simulink model "OpenAUV_v1dist"  (R2025a)
settings: Solver=VariableStepAuto  StartTime=0.0  StopTime=80  RelTol=1e-3
InitFcn:
  | initialization
values from neighbouring files (symbols this model uses):
  cf_backward = 2.9e-5    (= 2.9e-05)    [initialization.m]
  cf_forward = 4.7e-5    (= 4.7e-05)    [initialization.m]
  D_L = diag([5.9341, 4.3172, 6.2491, 0.0199, 0.4611, 0.0698])    [initialization.m]
  D_Q = diag([19.374, 42.687, 51.0402, 0.0668, 1.9172, 1.1343])    [initialization.m]
  Delta = M / rho    (= 0.0185)    [initialization.m]
  g = 9.81    [initialization.m]
  Ib = diag([0.3432, 1.4483, 1.5047]) + Ib_added    [initialization.m]
  lin_vel_0 = [dot_x0 dot_y0 dot_z0]    [initialization.m]
  mass = M * eye(3) + M_a    [initialization.m]
  pos_0 = [x0 y0 z0]    [initialization.m]
  r_b_b = [-0.2; 0; 0.2]    [initialization.m]
  r_c_b = [0; 0; 0]    [initialization.m]
  rho = 1000    [initialization.m]
  Ts = 0.001    [initialization.m]
  w_bb_0 = [0 0 0]    [initialization.m]
undefined symbols (not defined in the file or in its folder): DiscIntNeverNeededParam
libraries: matrix_library x1
settings Model: Creator=fabioruggiero  LastModifiedBy=Acer
settings ModelReferenceCC: EnableRefExpFcnMdlSchedulingChecks=on
settings RTWCC: GPUComputeCapability=3.5

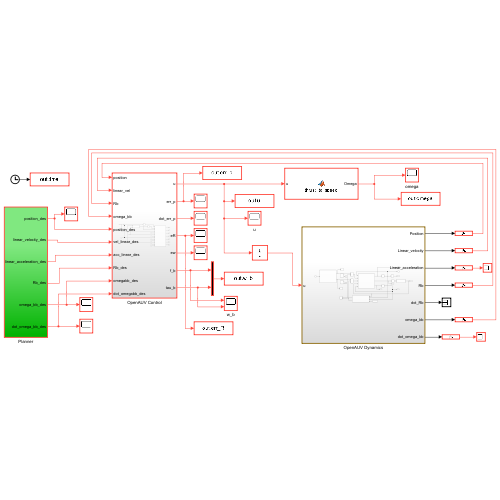
[thumbnail: Simulink's stored preview of the top-level diagram]
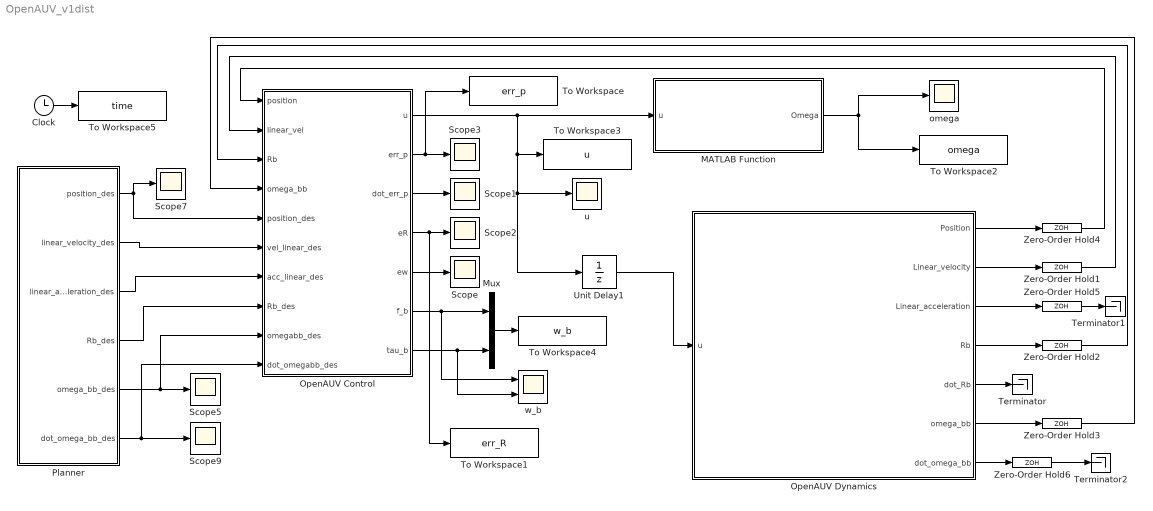
== system OpenAUV_v1dist ==
  Clock : Clock
  MATLAB Function : MATLAB Function  TreatAsAtomicUnit=on
  Mux : Mux  Inputs=2
  OpenAUV Control : Subsystem
  OpenAUV Dynamics : Subsystem
  Planner : Subsystem
  Scope{,1..3,5,7,9} (7 alike) : Scope
      Scope settings: Title=Angular Velocity errors  ActiveDisplayYMinimum=-1  ActiveDisplayYMaximum=1  YLabel=rad/s
      Scope1 settings: Title=Linear Velocity errors  ActiveDisplayYMinimum=-0.042668  ActiveDisplayYMaximum=0.038422  YLabel=m/s
      Scope2 settings: Title=Orientation error  ActiveDisplayYMinimum=-0.013334  ActiveDisplayYMaximum=0.012271
      Scope3 settings: Title=Position errors  ActiveDisplayYMinimum=-0.050218  ActiveDisplayYMaximum=0.073227  YLabel=m  DataLoggingVariableName=ScopeData2
      Scope5 settings: ActiveDisplayYMinimum=-0.15883  ActiveDisplayYMaximum=0.31625
      Scope7 settings: ActiveDisplayYMinimum=-4.625  ActiveDisplayYMaximum=1.625  DataLoggingVariableName=ScopeData2
      Scope9 settings: ActiveDisplayYMinimum=-0.05769  ActiveDisplayYMaximum=0.05769  DataLoggingVariableName=ScopeData2
  Terminator : Terminator
  Terminator1 : Terminator
  Terminator2 : Terminator
  To Workspace : ToWorkspace  VariableName=err_p  SaveFormat=Structure With Time  SampleTime=-1
  To Workspace1 : ToWorkspace  VariableName=err_R  SaveFormat=Structure With Time  SampleTime=-1
  To Workspace2 : ToWorkspace  VariableName=omega  SaveFormat=Structure With Time  SampleTime=-1
  To Workspace3 : ToWorkspace  VariableName=u  SaveFormat=Structure With Time  SampleTime=-1
  To Workspace4 : ToWorkspace  VariableName=w_b  SaveFormat=Structure With Time  SampleTime=-1
  To Workspace5 : ToWorkspace  VariableName=time  SaveFormat=Structure With Time  SampleTime=Ts
  Unit Delay1 : UnitDelay  InitialCondition=1.952815847891130e+05*ones(8,1)  SampleTime=-1
  Zero-Order Hold{1..6} (6 alike) : ZeroOrderHold  SampleTime=Ts
  omega : Scope
      settings: ActiveDisplayYMinimum=-1  ActiveDisplayYMaximum=1  DataLoggingVariableName=ScopeData3
  u : Scope
      settings: Title=u_w  ActiveDisplayYMinimum=-266.6856  ActiveDisplayYMaximum=244.3929  DataLoggingVariableName=ScopeData4
  w_b : Scope  NumInputPorts=2
      settings: Title=Control Forces  ActiveDisplayYMinimum=-17.0005  ActiveDisplayYMaximum=23.0413  YLabel=N
  wires:
  OpenAUV Dynamics/1(Position) -> Zero-Order Hold4/1
  OpenAUV Dynamics/2(Linear_velocity) -> Zero-Order Hold1/1
  OpenAUV Dynamics/4(Rb) -> Zero-Order Hold2/1
  OpenAUV Dynamics/6(omega_bb) -> Zero-Order Hold3/1
  Zero-Order Hold4/1 -> OpenAUV Control/1(position)
  OpenAUV Dynamics/5(dot_Rb) -> Terminator/1
  Planner/1(position_des) -> OpenAUV Control/5(position_des), Scope7/1
  OpenAUV Dynamics/3(Linear_acceleration) -> Zero-Order Hold5/1
  OpenAUV Dynamics/7(dot_omega_bb) -> Zero-Order Hold6/1
  Unit Delay1/1 -> OpenAUV Dynamics/1(u)
  Planner/4(Rb_des) -> OpenAUV Control/8(Rb_des)
  Planner/5(omega_bb_des) -> OpenAUV Control/9(omegabb_des), Scope5/1
  Planner/6(dot_omega_bb_des) -> OpenAUV Control/10(dot_omegabb_des), Scope9/1
  Zero-Order Hold5/1 -> Terminator1/1
  Zero-Order Hold6/1 -> Terminator2/1
  Mux/1 -> To Workspace4/1
  OpenAUV Control/7(tau_b) -> w_b/2, Mux/2
  OpenAUV Control/6(f_b) -> w_b/1, Mux/1
  OpenAUV Control/4(eR) -> To Workspace1/1, Scope2/1
  OpenAUV Control/2(err_p) -> Scope3/1, To Workspace/1
  Zero-Order Hold1/1 -> OpenAUV Control/2(linear_vel)
  Zero-Order Hold2/1 -> OpenAUV Control/3(Rb)
  Zero-Order Hold3/1 -> OpenAUV Control/4(omega_bb)
  Planner/2(linear_velocity_des) -> OpenAUV Control/6(vel_linear_des)
  Planner/3(linear_acceleration_des) -> OpenAUV Control/7(acc_linear_des)
  OpenAUV Control/3(dot_err_p) -> Scope1/1
  OpenAUV Control/5(ew) -> Scope/1
  Clock/1 -> To Workspace5/1
  MATLAB Function/1(Omega) -> To Workspace2/1, omega/1
  OpenAUV Control/1(u) -> MATLAB Function/1(u), Unit Delay1/1, u/1, To Workspace3/1

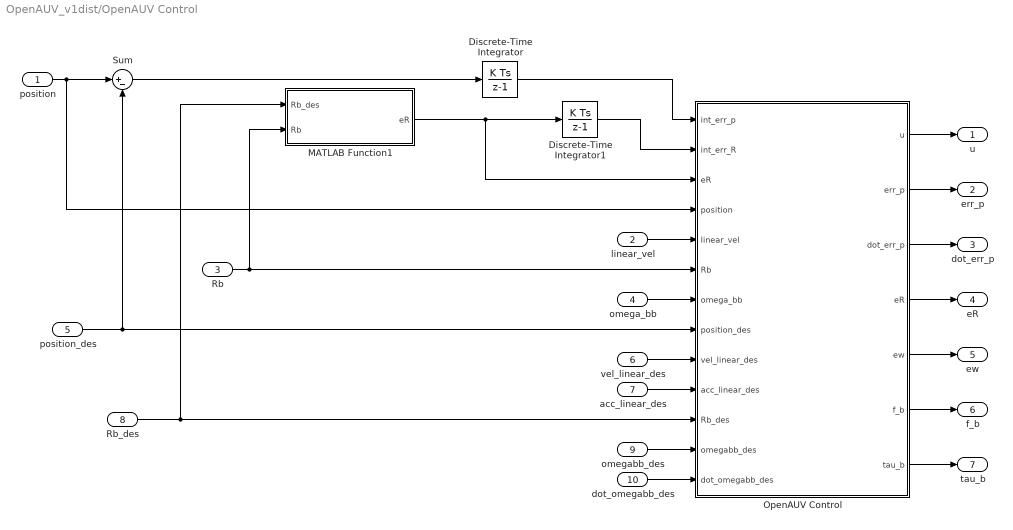
== system OpenAUV_v1dist/OpenAUV Control ==
  position : Inport
  linear_vel : Inport  Port=2
  Rb : Inport  Port=3
  omega_bb : Inport  Port=4
  position_des : Inport  Port=5
  vel_linear_des : Inport  Port=6
  acc_linear_des : Inport  Port=7
  Rb_des : Inport  Port=8
  omegabb_des : Inport  Port=9
  dot_omegabb_des : Inport  Port=10
  Discrete-Time Integrator : DiscreteIntegrator  SampleTime=Ts  UpperSaturationLimit=1.44  LowerSaturationLimit=-1.44  ICPrevOutput=DiscIntNeverNeededParam  ICPrevScaledInput=DiscIntNeverNeededParam
  Discrete-Time Integrator1 : DiscreteIntegrator  SampleTime=Ts  UpperSaturationLimit=1.44  LowerSaturationLimit=-1.44  ICPrevOutput=DiscIntNeverNeededParam  ICPrevScaledInput=DiscIntNeverNeededParam
  MATLAB Function1 : MATLAB Function  TreatAsAtomicUnit=on
  OpenAUV Control : MATLAB Function  TreatAsAtomicUnit=on
  Sum : Sum  Inputs=|+-
  u : Outport
  err_p : Outport  Port=2
  dot_err_p : Outport  Port=3
  eR : Outport  Port=4
  ew : Outport  Port=5
  f_b : Outport  Port=6
  tau_b : Outport  Port=7
  wires:
  OpenAUV Control/2(err_p) -> err_p/1
  vel_linear_des/1 -> OpenAUV Control/9(vel_linear_des)
  OpenAUV Control/3(dot_err_p) -> dot_err_p/1
  acc_linear_des/1 -> OpenAUV Control/10(acc_linear_des)
  OpenAUV Control/5(ew) -> ew/1
  dot_omegabb_des/1 -> OpenAUV Control/13(dot_omegabb_des)
  OpenAUV Control/4(eR) -> eR/1
  omegabb_des/1 -> OpenAUV Control/12(omegabb_des)
  OpenAUV Control/1(u) -> u/1
  Rb_des/1 -> MATLAB Function1/1(Rb_des), OpenAUV Control/11(Rb_des)
  position_des/1 -> Sum/2, OpenAUV Control/8(position_des)
  Sum/1 -> Discrete-Time Integrator/1
  MATLAB Function1/1(eR) -> OpenAUV Control/3("eR "), Discrete-Time Integrator1/1
  Discrete-Time Integrator/1 -> OpenAUV Control/1(int_err_p)
  Discrete-Time Integrator1/1 -> OpenAUV Control/2(int_err_R)
  position/1 -> OpenAUV Control/4(position), Sum/1
  linear_vel/1 -> OpenAUV Control/5(linear_vel)
  Rb/1 -> MATLAB Function1/2(Rb), OpenAUV Control/6(Rb)
  omega_bb/1 -> OpenAUV Control/7(omega_bb)
  OpenAUV Control/6(f_b) -> f_b/1
  OpenAUV Control/7(tau_b) -> tau_b/1

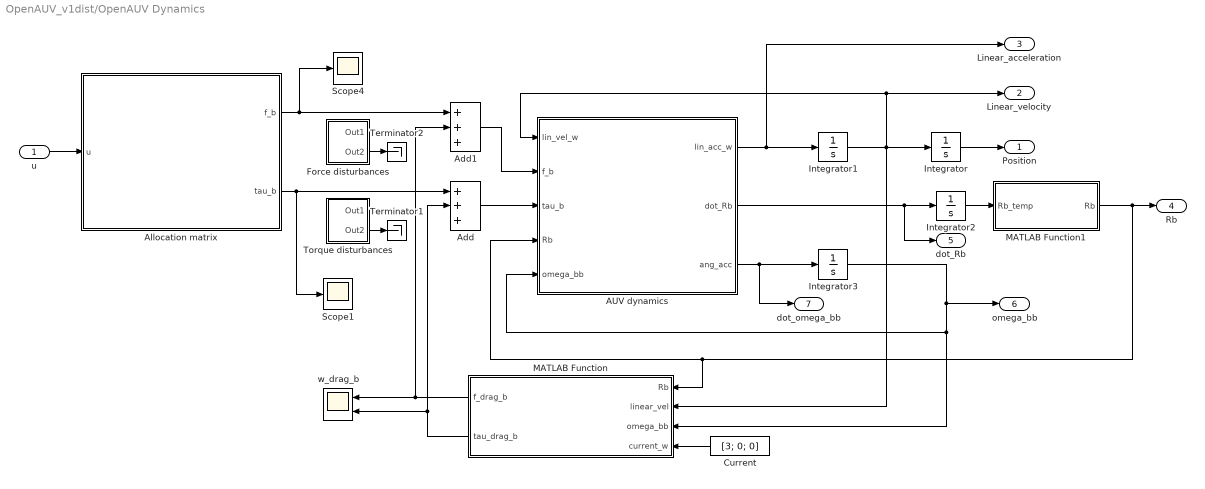
== system OpenAUV_v1dist/OpenAUV Dynamics ==
  u : Inport
  AUV dynamics : MATLAB Function  TreatAsAtomicUnit=on
  Add : Sum  Inputs=+++
  Add1 : Sum  Inputs=+++
  Allocation matrix : MATLAB Function  TreatAsAtomicUnit=on
  Current : Constant  Value=[3; 0; 0]
  Force disturbances : Subsystem
  Integrator : Integrator  InitialCondition=pos_0
  Integrator1 : Integrator  InitialCondition=lin_vel_0
  Integrator2 : Integrator  InitialCondition=[1 0 0; 0 1 0;0 0 1]
  Integrator3 : Integrator  InitialCondition=w_bb_0
  MATLAB Function : MATLAB Function  TreatAsAtomicUnit=on
  MATLAB Function1 : MATLAB Function  TreatAsAtomicUnit=on
  Scope1 : Scope
      settings: ActiveDisplayYMinimum=59.5491  ActiveDisplayYMaximum=72.8634  DataLoggingVariableName=ScopeData5
  Scope4 : Scope
      settings: ActiveDisplayYMinimum=-313.8933  ActiveDisplayYMaximum=214.6097  DataLoggingVariableName=ScopeData4
  Terminator1 : Terminator
  Terminator2 : Terminator
  Torque disturbances : Subsystem
  w_drag_b : Scope  NumInputPorts=2
      settings: Title=f_drag_b  ActiveDisplayYMinimum=-0.27226  ActiveDisplayYMaximum=1.5303  YLabel=N
  Position : Outport
  Linear_velocity : Outport  Port=2
  Linear_acceleration : Outport  Port=3
  Rb : Outport  Port=4
  dot_Rb : Outport  Port=5
  omega_bb : Outport  Port=6
  dot_omega_bb : Outport  Port=7
  wires:
  Integrator/1 -> Position/1
  AUV dynamics/3(ang_acc) -> dot_omega_bb/1, Integrator3/1
  Integrator3/1 -> MATLAB Function/3(omega_bb), AUV dynamics/5(omega_bb), omega_bb/1
  AUV dynamics/2(dot_Rb) -> dot_Rb/1, Integrator2/1
  MATLAB Function1/1(Rb) -> Rb/1, MATLAB Function/1(Rb), AUV dynamics/4(Rb)
  Integrator2/1 -> MATLAB Function1/1(Rb_temp)
  u/1 -> Allocation matrix/1(u)
  AUV dynamics/1(lin_acc_w) -> Linear_acceleration/1, Integrator1/1
  Add/1 -> AUV dynamics/3(tau_b)
  Add1/1 -> AUV dynamics/2(f_b)
  MATLAB Function/1(f_drag_b) -> w_drag_b/1, Add1/2
  MATLAB Function/2(tau_drag_b) -> w_drag_b/2, Add/2
  Current/1 -> MATLAB Function/4(current_w)
  Integrator1/1 -> Integrator/1, MATLAB Function/2(linear_vel), Linear_velocity/1, AUV dynamics/1(lin_vel_w)
  Allocation matrix/2(tau_b) -> Add/1, Scope1/1
  Allocation matrix/1(f_b) -> Scope4/1, Add1/1
  Force disturbances/2(Out2) -> Terminator2/1
  Torque disturbances/2(Out2) -> Terminator1/1

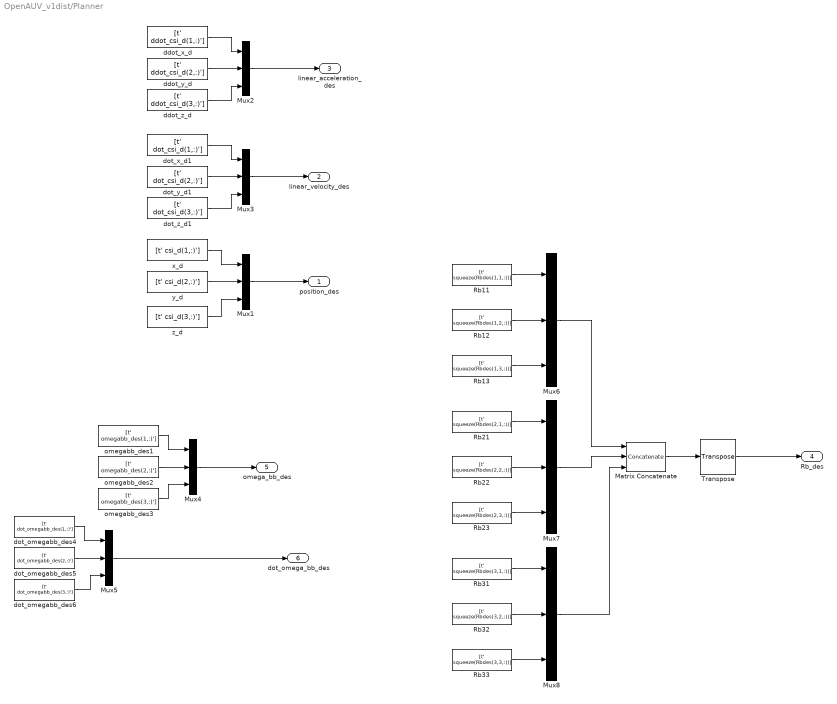
== system OpenAUV_v1dist/Planner ==
  Matrix Concatenate : Concatenate  NumInputs=3  Mode=Multidimensional array  ConcatenateDimension=2
  Mux{1..8} (8 alike) : Mux  Inputs=3
  Rb11 : FromWorkspace  VariableName=[t' squeeze(Rbdes(1,1,:))]  SampleTime=Ts
  Rb12 : FromWorkspace  VariableName=[t' squeeze(Rbdes(1,2,:))]  SampleTime=Ts
  Rb13 : FromWorkspace  VariableName=[t' squeeze(Rbdes(1,3,:))]  SampleTime=Ts
  Rb21 : FromWorkspace  VariableName=[t' squeeze(Rbdes(2,1,:))]  SampleTime=Ts
  Rb22 : FromWorkspace  VariableName=[t' squeeze(Rbdes(2,2,:))]  SampleTime=Ts
  Rb23 : FromWorkspace  VariableName=[t' squeeze(Rbdes(2,3,:))]  SampleTime=Ts
  Rb31 : FromWorkspace  VariableName=[t' squeeze(Rbdes(3,1,:))]  SampleTime=Ts
  Rb32 : FromWorkspace  VariableName=[t' squeeze(Rbdes(3,2,:))]  SampleTime=Ts
  Rb33 : FromWorkspace  VariableName=[t' squeeze(Rbdes(3,3,:))]  SampleTime=Ts
  Transpose : matrix_library/Transpose
  ddot_x_d : FromWorkspace  VariableName=[t' ddot_csi_d(1,:)']  SampleTime=Ts
  ddot_y_d : FromWorkspace  VariableName=[t' ddot_csi_d(2,:)']  SampleTime=Ts
  ddot_z_d : FromWorkspace  VariableName=[t' ddot_csi_d(3,:)']  SampleTime=Ts
  dot_omegabb_des4 : FromWorkspace  VariableName=[t' dot_omegabb_des(1,:)']  SampleTime=Ts
  dot_omegabb_des5 : FromWorkspace  VariableName=[t' dot_omegabb_des(2,:)']  SampleTime=Ts
  dot_omegabb_des6 : FromWorkspace  VariableName=[t' dot_omegabb_des(3,:)']  SampleTime=Ts
  dot_x_d1 : FromWorkspace  VariableName=[t' dot_csi_d(1,:)']  SampleTime=Ts
  dot_y_d1 : FromWorkspace  VariableName=[t' dot_csi_d(2,:)']  SampleTime=Ts
  dot_z_d1 : FromWorkspace  VariableName=[t' dot_csi_d(3,:)']  SampleTime=Ts
  omegabb_des1 : FromWorkspace  VariableName=[t' omegabb_des(1,:)']  SampleTime=Ts
  omegabb_des2 : FromWorkspace  VariableName=[t' omegabb_des(2,:)']  SampleTime=Ts
  omegabb_des3 : FromWorkspace  VariableName=[t' omegabb_des(3,:)']  SampleTime=Ts
  x_d : FromWorkspace  VariableName=[t' csi_d(1,:)']  SampleTime=Ts
  y_d : FromWorkspace  VariableName=[t' csi_d(2,:)']  SampleTime=Ts
  z_d : FromWorkspace  VariableName=[t' csi_d(3,:)']  SampleTime=Ts
  position_des : Outport
  linear_velocity_des : Outport  Port=2
  linear_acceleration_des : Outport  Port=3
  Rb_des : Outport  Port=4
  omega_bb_des : Outport  Port=5
  dot_omega_bb_des : Outport  Port=6
  wires:
  y_d/1 -> Mux1/2
  z_d/1 -> Mux1/3
  x_d/1 -> Mux1/1
  ddot_y_d/1 -> Mux2/2
  ddot_z_d/1 -> Mux2/3
  ddot_x_d/1 -> Mux2/1
  Mux2/1 -> linear_acceleration_des/1
  Mux1/1 -> position_des/1
  dot_y_d1/1 -> Mux3/2
  dot_z_d1/1 -> Mux3/3
  dot_x_d1/1 -> Mux3/1
  Mux3/1 -> linear_velocity_des/1
  Mux5/1 -> dot_omega_bb_des/1
  omegabb_des3/1 -> Mux4/3
  Mux4/1 -> omega_bb_des/1
  omegabb_des2/1 -> Mux4/2
  omegabb_des1/1 -> Mux4/1
  dot_omegabb_des4/1 -> Mux5/1
  dot_omegabb_des5/1 -> Mux5/2
  dot_omegabb_des6/1 -> Mux5/3
  Rb11/1 -> Mux6/1
  Rb12/1 -> Mux6/2
  Rb13/1 -> Mux6/3
  Rb23/1 -> Mux7/3
  Rb22/1 -> Mux7/2
  Rb21/1 -> Mux7/1
  Rb31/1 -> Mux8/1
  Rb32/1 -> Mux8/2
  Rb33/1 -> Mux8/3
  Mux6/1 -> Matrix Concatenate/1
  Mux7/1 -> Matrix Concatenate/2
  Mux8/1 -> Matrix Concatenate/3
  Matrix Concatenate/1 -> Transpose/1
  Transpose/1 -> Rb_des/1

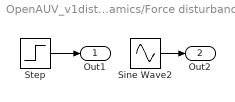
== system OpenAUV_v1dist/OpenAUV Dynamics/Force disturbances ==
  Sine Wave2 : Sin  Amplitude=8  Frequency=0.5  SampleTime=0
  Step : Step  Time=4  After=1.5  SampleTime=0
  Out1 : Outport
  Out2 : Outport  Port=2
  wires:
  Sine Wave2/1 -> Out2/1
  Step/1 -> Out1/1

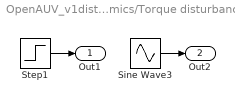
== system OpenAUV_v1dist/OpenAUV Dynamics/Torque disturbances ==
  Sine Wave3 : Sin  Amplitude=2  Frequency=0.5  SampleTime=0
  Step1 : Step  Time=4  After=1.5  SampleTime=0
  Out1 : Outport
  Out2 : Outport  Port=2
  wires:
  Sine Wave3/1 -> Out2/1
  Step1/1 -> Out1/1

== matlab function OpenAUV_v1dist/OpenAUV Control/MATLAB Function1 ==
  data: Rb_des input; eR output; Rb input
function eR = orientation_error(Rb_des, Rb)
eR = 0.5 * vee(Rb_des' * Rb - Rb' * Rb_des);
end

function v = vee(S)
v = [S(3,2); S(1,3); S(2,1)];
end

== matlab function OpenAUV_v1dist/OpenAUV Dynamics/MATLAB Function1 ==
  data: Rb_temp input; Rb output
function Rb = fcn(Rb_temp)
    [U,S,V] = svd(Rb_temp);
    sigma = det(U*V');
    S_ = diag([1 1 sigma]);

    Rb = U*S_*V';
end

== matlab function OpenAUV_v1dist/OpenAUV Dynamics/MATLAB Function ==
  data: Rb input; f_drag_b output; linear_vel input; tau_drag_b output; omega_bb input; current_w input
function [f_drag_b, tau_drag_b] = drag_disturbance(Rb, linear_vel, omega_bb, current_w)
% wind_w: Wind velocity vector in the inertial frame [m/s]

% 1. Compute the RELATIVE VELOCITY of the AUV with respect to the ocean current in the inertial frame
linear_vel_rel_w = linear_vel - current_w;

% 2. Transform the relative linear velocity into the body-fixed frame
vel_linear_rel_b = Rb' * linear_vel_rel_w; 

% 3. Define the Quadratic Drag matrices
Dv = diag([0.15, 0.15, 0.25]);   % Linear drag coefficients in the body frame
Dw = diag([0.02, 0.02, 0.04]);   % Rotational drag coefficients (independent of linear current)

% 4. Compute the forces in the body frame based on the RELATIVE velocity
% Note: the negative sign ensures that the drag force opposes the relative current velocity
f_drag_b = -Dv * vel_linear_rel_b * norm(vel_linear_rel_b);

% Rotational drag torques depend solely on the vehicle's own angular velocity
tau_drag_b = -Dw * omega_bb * norm(omega_bb);
end

== matlab function OpenAUV_v1dist/MATLAB Function ==
  data: u input; Omega output; cf_forward parameter; cf_backward parameter
function Omega = thrust_to_speed(u, cf_forward, cf_backward)

% Initialize the output vector
Omega = zeros(8, 1);

% 2. Map each force to its corresponding speed
for i = 1:8
    force = u(i);
    
    if force >= 0
        % Forward thrust: use highly efficient forward coefficient
        Omega(i) = sqrt(force / cf_forward);
    else
        % Backward thrust: use reduced backward coefficient and force negative sign
        Omega(i) = -sqrt(abs(force) / cf_backward);
    end
end

== matlab function OpenAUV_v1dist/OpenAUV Dynamics/Allocation matrix ==
  data: u input size=8; f_b output size=3; tau_b output size=3
function [f_b,tau_b] = allocation(u)

%% 1. OpenAUV Constant Thruster Configuration Matrix B (6 x 8)
B = [ 0.7071    0.7071   -0.7071   -0.7071         0         0         0         0;
      0.7071   -0.7071    0.7071   -0.7071         0         0         0         0;
           0         0         0         0    1.0000   -1.0000   -1.0000    1.0000;
           0         0         0         0    0.1300    0.1300   -0.1300   -0.1300;
           0         0         0         0   -0.2350    0.2350   -0.2350    0.2350;
      0.1485   -0.1485   -0.1485    0.1485         0         0         0         0];

%% 2. Compute Total Force and Torque
% Forward mapping using matrix multiplication: Wrench = B * u
wrench_b = B * u;

% Extract forces (Surge, Sway, Heave)
f_b = wrench_b(1:3);

% Extract torques (Roll, Pitch, Yaw)
tau_b = wrench_b(4:6);

end

== matlab function OpenAUV_v1dist/OpenAUV Dynamics/AUV dynamics ==
  data: lin_vel_w input; f_b input size=3; tau_b input size=3; Rb input size=[3,3]; omega_bb input size=3; mass parameter size=[3,3]; Ib parameter size=[3,3]; D_L parameter size=[6, 6]; D_Q parameter size=[6, 6]; lin_acc_w output size=3; dot_Rb output size=[3,3]; ang_acc output size=3; rho parameter; Delta parameter; g parameter; e3 parameter; r_c_b parameter; r_b_b parameter
function [lin_acc_w, dot_Rb, ang_acc] = fcn(lin_vel_w, f_b, tau_b, Rb, omega_bb, mass, Ib, D_L, D_Q, rho, Delta, g, e3, r_c_b, r_b_b)

%% 1. Frame Transformation for Linear Velocity
% Transform linear velocity vector from World frame to Body frame
lin_vel_b = Rb' * lin_vel_w;

%% 2. Drag Partitioning
% Extract diagonal 3x3 blocks from 6x6 linear and quadratic damping matrices
D_Lv = D_L(1:3, 1:3); D_Lw = D_L(4:6, 4:6);
D_Qv = D_Q(1:3, 1:3); D_Qw = D_Q(4:6, 4:6);

% Compute total linear and angular hydrodynamic damping vectors in Body frame
Dv_b = (D_Lv + D_Qv .* norm(lin_vel_b)) * lin_vel_b;
Dw_b = (D_Lw + D_Qw .* norm(omega_bb)) * omega_bb;

%% 3. Hydrostatic Forces and Moments (In Body Frame)
M = 18.5; % Dry mass from the vehicle datasheet
f_g_b = M * g * Rb' * e3;              % Gravity force vector projected into Body frame
f_b_b = - rho*Delta*g * Rb' * e3;      % Buoyancy force vector projected into Body frame
g_forces_b = - f_g_b - f_b_b;          % Net hydrostatic forces acting on the vehicle
g_torques_b = -skew(r_c_b)*f_g_b - skew(r_b_b)*f_b_b; % Net hydrostatic moments due to COG/COB offsets

%% 4. Net External Forces and Moments Evaluation (Body Frame)

% Compute the net total torque vector (including the rigid body gyroscopic/Coriolis term)
C_forces = skew(omega_bb) * (mass * lin_vel_b);
C_torques = skew(omega_bb) * (Ib * omega_bb) + skew(lin_vel_b) * (mass * lin_vel_b);

% Compute the net total force vector acting in the Body frame
F_net_b = f_b - Dv_b - g_forces_b - C_forces;
T_net_b = tau_b - Dw_b - g_torques_b - C_torques;

%% 5. Simultaneous Resolution of the Coupled System (Mass + Center of Gravity Offset)
% Position vector of the Center of Gravity (COG) in the Body frame
r_g = [0; 0; 0.02]; % Update this vector with the actual AUV value if different
S_rg = skew(r_g);

% Define the precise off-diagonal blocks of the rigid body inertia matrix M_RB
M_off1 = - M * S_rg; % Upper-right block (-m*S(rg))
M_off2 =   M * S_rg; % Lower-left block (m*S(rg))

% Matrix block inversion via Schur Complement method to solve the coupled 6DoF system:
% 'mass' is the 3x3 matrix combining rigid body mass and linear added mass
% 'Ib' is the 3x3 matrix combining rigid body inertia and angular added mass
Ib_eff = Ib - M_off2 * (mass \ M_off1);
T_eff  = T_net_b - M_off2 * (mass \ F_net_b);

% A. Exact computation of the angular acceleration in the Body frame
ang_acc = Ib_eff \ T_eff;

% B. Exact computation of the linear acceleration in the Body frame
lin_acc_b = mass \ (F_net_b - M_off1 * ang_acc);

%% 6. Final Transformation of Linear Acceleration into the World Frame
% This step ensures full compatibility with the external Simulink integrator (1/s),
% which operates in the World frame to evaluate global X, Y, Z positions.
lin_acc_w = Rb * lin_acc_b;

%% 7. Kinematics
% Time derivative of the rotation matrix based on angular velocity
dot_Rb = Rb * skew(omega_bb);

end

function S = skew(v)
if(numel(v) ~= 1)
    S = [0 -v(3) v(2); 
         v(3) 0 -v(1);
        -v(2) v(1) 0];
else
    S = zeros(3);
end
end

== matlab function OpenAUV_v1dist/OpenAUV Control/OpenAUV Control ==
  data: int_err_p input; int_err_R input; eR input; position input size=3; u output size=8; linear_vel input size=3; Rb input size=[3,3]; omega_bb input size=3; position_des input size=3; vel_linear_des input size=3; acc_linear_des input size=3; Rb_des input size=[3,3]; omegabb_des input; dot_omegabb_des input; err_p output size=3; dot_err_p output size=3; eR output size=3; ew output size=3; mass parameter; Ib parameter; f_b output; tau_b output; rho parameter; g parameter; r_c_b parameter; r_b_b parameter; Delta parameter; e3 parameter
function [u, err_p, dot_err_p, eR, ew, f_b, tau_b] = OpenAUV_control(int_err_p, int_err_R, eR, position, linear_vel, Rb, omega_bb, position_des, vel_linear_des, acc_linear_des, Rb_des, omegabb_des, dot_omegabb_des, ...
    mass, Ib, rho, g, r_c_b, r_b_b, Delta, e3)

%% 1. Gain Tuning (Standard Stable Values)
% Control loop parameter definition based on natural frequency (wn) and damping ratio (zeta)
wn_att = 1.2;
zeta_att = 0.8;
wn_pos = 0.8;
zeta_pos = zeta_att;

% Compute proportional, derivative, and integral gain matrices for position and attitude loops
Kp = wn_pos^2 * eye(3);
Kd = 2 * zeta_pos * wn_pos * eye(3);
KR = wn_att^2 * eye(3);
Kw = 2 * zeta_att * wn_att * eye(3);
Ki = 0.1 * eye(3);
KiR = 0.1 * eye(3);
% KiR = 0.7 * eye(3);

%% 2. Hydrodynamic Drag in BODY Frame
% D_L and D_Q represent 6x6 linear and quadratic damping coefficient matrices
D_L = diag([5.9341, 4.3172, 6.2491, 0.0199, 0.4611, 0.0698]);
D_Q = diag([19.374, 42.687, 51.0402, 0.0668, 1.9172, 1.1343]);

% Extract diagonal 3x3 blocks for uncoupled linear and angular damping evaluation
D_Lv = D_L(1:3, 1:3); D_Lw = D_L(4:6, 4:6);
D_Qv = D_Q(1:3, 1:3); D_Qw = D_Q(4:6, 4:6);

% Transform linear velocity vector from World frame to Body frame
linear_vel_b = Rb' * linear_vel;

% Compute linear and angular hydrodynamic damping force and torque vectors
Dv = (D_Lv + D_Qv .* norm(linear_vel_b)) * linear_vel_b;
Dw = (D_Lw + D_Qw .* norm(omega_bb)) * omega_bb;

%% 3. Hydrostatic Forces and Moments 
M = 18.5; % Dry mass evaluated for gravity force compensation
f_g_b = M * g * Rb' * e3;                    % Gravity force vector in Body frame
f_b_b = - rho * Delta * g * Rb' * e3;        % Buoyancy force vector in Body frame
g_forces_b = - f_g_b - f_b_b;                % Net hydrostatic restoring forces
g_torques_b = -skew(r_c_b)*f_g_b - skew(r_b_b)*f_b_b; % Net hydrostatic restoring torques due to COG/COB offsets

%% 4. Position Error Calculation (World Frame)
% Compute tracking errors for position and linear velocity
err_p = position - position_des;
dot_err_p = linear_vel - vel_linear_des; 

%% 5. Linear Feedback Linearization (Force Control f_b)
% Compute the virtual PID-based acceleration command in the World frame
acc_PID_w = acc_linear_des - Kp*err_p - Kd*dot_err_p - Ki*int_err_p;

% Project the desired virtual acceleration command into the vehicle Body frame
acc_PID_b = Rb' * acc_PID_w;

% Compute the complete Coriolis and Centripetal terms to be canceled (Rigid Body + Added Mass)
C_forces = skew(omega_bb) * (mass * linear_vel_b);
C_torques = skew(omega_bb) * (Ib * omega_bb) + skew(linear_vel_b) * (mass * linear_vel_b);

%% 6. Angular Velocity Error Calculation
% Compute tracking error for angular velocity in the Body frame
ew = omega_bb - Rb' * Rb_des * omegabb_des;

%% 7. Rotational Feedback Linearization (Torque Control tau_b)
% Compute desired orientation feedforward parameters in the Body frame
omega_des_b = Rb' * Rb_des * omegabb_des;
dot_omega_des_b = Rb' * Rb_des * dot_omegabb_des;

% Compute the virtual geometric tracking acceleration command incorporating feedforward terms
ang_acc_PID = - KR*eR - Kw*ew - KiR*int_err_R - skew(omega_bb)*omega_des_b + dot_omega_des_b;

%% --- CENTER OF GRAVITY CORRECTION TERMS (Reference Matrix M_RB) ---
% Position vector of the Center of Gravity (COG) in the Body frame
r_g = [0; 0; 0.02]; % Center of Gravity position vector
S_rg = skew(r_g);

% Compute inertial off-diagonal coupling terms: -m*S(rg)*dot_omega and m*S(rg)*dot_v
f_coupling = - M * S_rg * ang_acc_PID;
tau_coupling = M * S_rg * acc_PID_b;

% Full Feedback Linearization control laws canceling inertia cross-coupling, damping, and hydrostatics
f_b = mass * acc_PID_b + f_coupling + Dv + g_forces_b + C_forces;
tau_b = Ib * ang_acc_PID + tau_coupling + Dw + g_torques_b + C_torques;

%% 8. Total Wrench & OpenAUV Static Allocation
% Group control forces and torques into the 6DoF body wrench vector
w_b = [f_b; tau_b];

% OpenAUV Constant Thruster Configuration Matrix B (6 x 8)
% Columns reflect positive thrust directions mapping validated from the vehicle physical layout
B = [ 0.7071    0.7071   -0.7071   -0.7071         0         0         0         0;
      0.7071   -0.7071    0.7071   -0.7071         0         0         0         0;
           0         0         0         0    1.0000   -1.0000   -1.0000    1.0000;
           0         0         0         0    0.1300    0.1300   -0.1300   -0.1300;
           0         0         0         0   -0.2350    0.2350   -0.2350    0.2350;
      0.1485   -0.1485   -0.1485    0.1485         0         0         0         0];

% Static control allocation via pseudo-inverse mapping directly to the 8 independent motors
u = pinv(B) * w_b;

end

function S = skew(v)
    if(numel(v) ~= 1)
        S = [0,    -v(3),  v(2); 
             v(3),  0,    -v(1);
            -v(2),  v(1),  0];
    else
        S = zeros(3);
    end
end
